simulink model "model2_22"  (R2020a)
settings: Solver=ode4  StartTime=0  StopTime=10  FixedStep=0.001  RelTol=1e-3
undefined symbols (not defined in the file): a1, a2, a3, a4, b, C, Data_Display, H, model2
libraries: androiduilib x2
settings Model: Creator=sebastian  LastModifiedBy=corte
settings OptimizationCC: EnhancedBackFolding=on  PassReuseOutputArgsAs=Individual arguments  ZeroExternalMemoryAtStartup=off  ZeroInternalMemoryAtStartup=off  MaxStackSize=64  OptimizeBlockOrder=speed  DifferentSizesBufferReuse=on  OptimizationCustomize=off  EfficientTunableParamExpr=on
settings DebuggingCC: ParameterTunabilityLossMsg=error
settings HardwareCC: ProdBitPerPointer=32  ProdBitPerSizeT=32  ProdBitPerPtrDiffT=32  ProdLargestAtomicInteger=Long  ProdLargestAtomicFloat=Double  ProdWordSize=32  ProdHWDeviceType=ARM Compatible->ARM Cortex
settings SFSimCC: MATLABDynamicMemAlloc=off
settings RTWCC: SystemTargetFile=ert.tlc  HardwareBoard=Android Device  TemplateMakefile=ert_default_tmf  RTWVerbose=off  Toolchain=Android SDK/NDK Tools
settings CodeAppCC: ForceParamTrailComments=on  IgnoreCustomStorageClasses=off  OperatorAnnotations=on  SimulinkDataObjDesc=on  SFDataObjDesc=on  InsertBlockDesc=on
settings ERTTargetCC: SupportContinuousTime=on

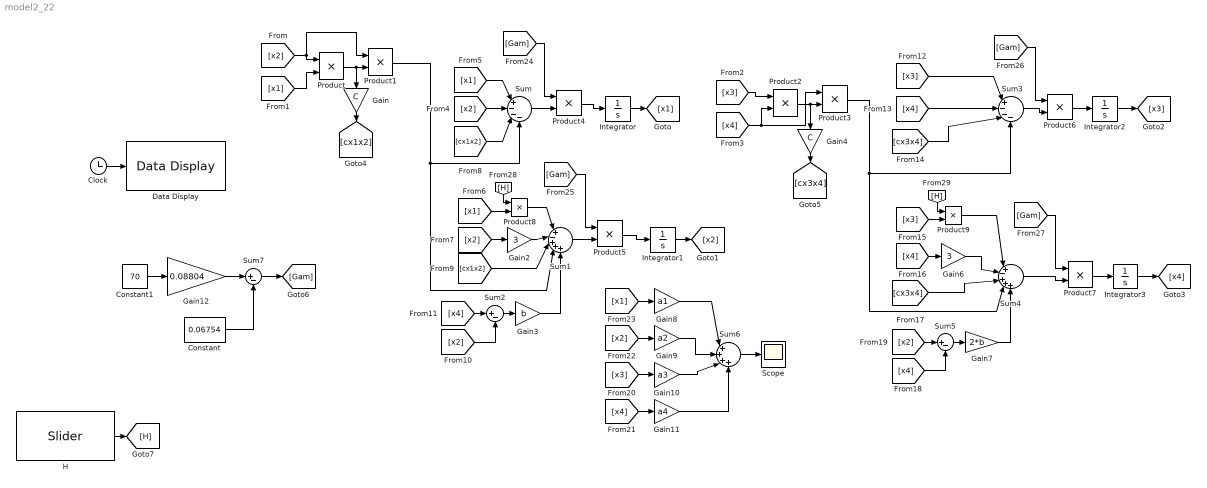
== system model2_22 ==
  Clock : Clock
  Constant : Constant  Value=0.06754
  Constant1 : Constant  Value=70
  Data Display : androiduilib/Data Display  DataDisplayId=model2/Data_Display  Format=Float  Precision=6  SimulateUsing=Code generation  blockPlatform=Android
      settings: SourceProductBaseCode=ANDROID
  Gain : Gain  Gain=C
  Gain10 : Gain  Gain=a3
  Gain11 : Gain  Gain=a4
  Gain12 : Gain  Gain=0.08804
  Gain2 : Gain  Gain=3
  Gain3 : Gain  Gain=b
  Gain4 : Gain  Gain=C
  Gain6 : Gain  Gain=3
  Gain7 : Gain  Gain=2*b
  Gain8 : Gain  Gain=a1
  Gain9 : Gain  Gain=a2
  H : androiduilib/Slider  Min=2  Value=3  Max=5  Resolution=0.1  SliderId=model2/H  SampleTime=0.05  BlockPlatform=Android
      settings: SourceProductBaseCode=ANDROID
  Integrator : Integrator
  Integrator1 : Integrator
  Integrator2 : Integrator  InitialCondition=0.1
  Integrator3 : Integrator
  Product{,1..9} (10 alike) : Product
  Scope : Scope
  Sum : Sum  Inputs=|+---
  Sum1 : Sum  Inputs=|+-+++
  Sum2 : Sum  Inputs=|+-
  Sum3 : Sum  Inputs=|+---
  Sum4 : Sum  Inputs=|+-+++
  Sum5 : Sum  Inputs=|+-
  Sum6 : Sum  Inputs=|++++
  Sum7 : Sum  Inputs=|+-
  wires:
  Integrator/1 -> [x1]
  Integrator1/1 -> [x2]
  Integrator2/1 -> [x3]
  Integrator3/1 -> [x4]
  [x2] -> Product/1, Product1/1
  [x1] -> Product/2
  Product/1 -> Gain/1, Product1/2
  Product2/1 -> Gain4/1, Product3/2
  [x3] -> Product2/1
  [x4] -> Product3/1, Product2/2
  [x2] -> Sum/2
  [x1] -> Sum/1
  Product1/1 -> Sum/4, Sum1/4
  Product8/1 -> Sum1/1
  [x1] -> Product8/2
  [x2] -> Gain2/1
  Gain2/1 -> Sum1/2
  Gain/1 -> [cx1x2]
  [cx1x2] -> Sum/3
  [cx1x2] -> Sum1/3
  Gain3/1 -> Sum1/5
  Sum2/1 -> Gain3/1
  [x4] -> Sum2/1
  [x2] -> Sum2/2
  Gain4/1 -> [cx3x4]
  [x3] -> Sum3/1
  [x4] -> Sum3/2
  [cx3x4] -> Sum3/3
  Product3/1 -> Sum3/4, Sum4/4
  [x3] -> Product9/2
  Product9/1 -> Sum4/1
  [x4] -> Gain6/1
  Gain6/1 -> Sum4/2
  [cx3x4] -> Sum4/3
  [x2] -> Sum5/1
  [x4] -> Sum5/2
  Sum5/1 -> Gain7/1
  Gain7/1 -> Sum4/5
  Gain8/1 -> Sum6/1
  Gain9/1 -> Sum6/2
  Gain10/1 -> Sum6/3
  Gain11/1 -> Sum6/4
  [x3] -> Gain10/1
  [x4] -> Gain11/1
  [x1] -> Gain8/1
  [x2] -> Gain9/1
  Sum6/1 -> Scope/1
  Sum/1 -> Product4/2
  Product4/1 -> Integrator/1
  Sum1/1 -> Product5/2
  Product5/1 -> Integrator1/1
  Sum3/1 -> Product6/2
  Product6/1 -> Integrator2/1
  Sum4/1 -> Product7/2
  Product7/1 -> Integrator3/1
  [Gam] -> Product4/1
  [Gam] -> Product5/1
  [Gam] -> Product6/1
  [Gam] -> Product7/1
  Constant1/1 -> Gain12/1
  Gain12/1 -> Sum7/1
  Sum7/1 -> [Gam]
  Constant/1 -> Sum7/2
  H/1 -> [H]
  [H] -> Product8/1
  [H] -> Product9/1
  Clock/1 -> Data Display/1
